simulink model "mainsimu1"  (Simulink 8.0)
settings: Solver=ode4  StartTime=0.0  StopTime=stop_time  FixedStep=step_time  RelTol=1e-3
values from neighbouring files (symbols this model uses):
  alpha = 0.2    [main_1.m]
  Exp_Lamda = 8.1    [main_1.m]
  mean_wind = 5    [main_1.m]
  R = 21.65    [main_1.m]
settings Model: Creator=Administrator  LastModifiedBy=dujiexian
settings DataIOCC: SignalLoggingSaveFormat=ModelDataLogs
settings DebuggingCC: CheckSSInitialOutputMsg=off  FcnCallInpInsideContextMsg=UseLocalSettings
settings GRTTargetCC: CombineOutputUpdateFcns=off  GRTInterface=on

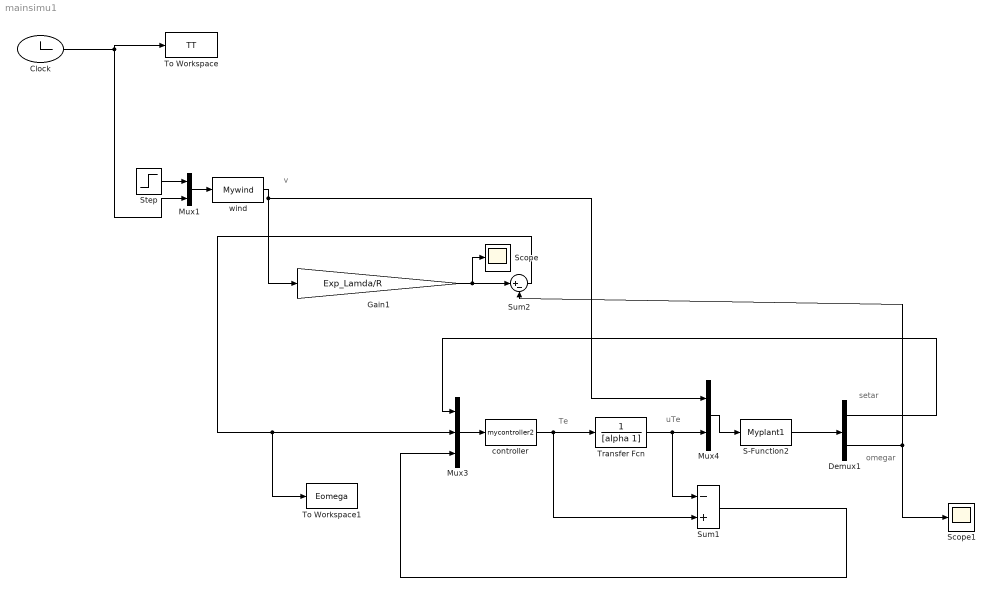
== system mainsimu1 ==
  note: v
  note: Te
  note: uTe
  note: setar
  note: omegar
  Clock : Clock
  Demux1 : Demux  Outputs=2
  Gain1 : Gain  Gain=Exp_Lamda/R
  Mux1 : Mux  Inputs=2
  Mux3 : Mux  Inputs=3
  Mux4 : Mux  Inputs=2
  S-Function2 : S-Function  FunctionName=Myplant1  EnableBusSupport=off
  Scope : Scope
      settings: YMin=2.25  YMax=2.675
  Scope1 : Scope
      settings: YMin=0.05225  YMax=0.0524
  Step : Step  Time=0  After=mean_wind  SampleTime=0
  Sum1 : Sum  Inputs=-+
  Sum2 : Sum  Inputs=|+-
  To Workspace : ToWorkspace  VariableName=TT  SampleTime=-1
  To Workspace1 : ToWorkspace  VariableName=Eomega  SampleTime=-1
  Transfer Fcn : TransferFcn  Denominator=[alpha 1]
  "controller " : MATLABFcn  MATLABFcn=mycontroller2
  wind : MATLABFcn  MATLABFcn=Mywind
  wires:
  Clock/1 -> To Workspace/1, Mux1/2
  Step/1 -> Mux1/1
  Mux1/1 -> wind/1
  "controller "/1 -> Transfer Fcn/1, Sum1/2
  S-Function2/1 -> Demux1/1
  Demux1/1 -> Mux3/1
  Demux1/2 -> Sum2/2, Scope1/1
  Mux3/1 -> "controller "/1
  wind/1 -> Gain1/1, Mux4/1
  Gain1/1 -> Sum2/1, Scope/1
  Sum2/1 -> Mux3/2, To Workspace1/1
  Transfer Fcn/1 -> Mux4/2, Sum1/1
  Mux4/1 -> S-Function2/1
  Sum1/1 -> Mux3/3
